simulink model "stm32f0_eep_emulation_demo"  (Simulink 7.3)
settings: Solver=FixedStepDiscrete  SolverMode=SingleTasking  StartTime=0.0  StopTime=10  RelTol=1e-3
PreLoadFcn:
  | waijung.modelPreload; % Required for working with Waijung Blockset. Do not remove.
undefined symbols (not defined in the file): LQFP48, STM32F072CB
libraries: simulink x1, stm32f0_device_config_lib x1
CloseFcn:
  | waijung.modelClose; % Required for working with Waijung Blockset. Do not remove.
settings Model: Creator=Krisada  LastModifiedBy=Krisada
settings OptimizationCC: OptimizeModelRefInitCode=on  LifeSpan=1
settings HardwareCC: ProdEndianess=LittleEndian  ProdHWDeviceType=ARM Compatible->Cortex - M0  TargetEndianess=LittleEndian  TargetHWDeviceType=ARM Compatible->Cortex - M0
settings RTWCC: SystemTargetFile=stm32f0.tlc  GenerateMakefile=off  TemplateMakefile=ert_default_tmf  Description=STM32F0 Target  ProcessScript=stm32f0_make_rtw_hook
settings CodeAppCC: IgnoreCustomStorageClasses=off
settings STFCustomTargetCC: ModelReferenceCompliant=off  CombineOutputUpdateFcns=on  ERTCustomFileBanners=on  SupportContinuousTime=off  SupportNonInlinedSFcns=off  SystemTargetFile=stm32f0.tlc
settings ERTTargetCC: MultiwordLength=2048  ModelReferenceCompliant=off  ParMdlRefBuildCompliant=off  CompOptLevelCompliant=off  ERTFirstTimeCompliant=off  ModelStepFunctionPrototypeControlCompliant=off  CPPClassGenCompliant=off  ExtModeMexFile=noextcomm  InlinedParameterPlacement=NonHierarchical  ERTSrcFileBannerTemplate=stm32f0_code_template.cgt  ERTHdrFileBannerTemplate=stm32f0_code_template.cgt  ERTDataSrcFileTemplate=stm32f0_code_template.cgt  ERTDataHdrFileTemplate=stm32f0_code_template.cgt  ERTCustomFileTemplate=stm32f0_file_process.tlc

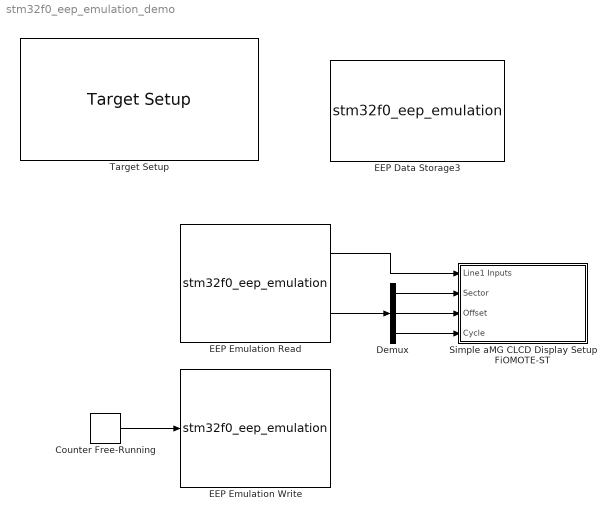
== system stm32f0_eep_emulation_demo ==
  Counter Free-Running : simulink/Sources/Counter Free-Running  SystemSampleTime=-1  NumBits=16  tsamp=-1
  Demux : Demux  Outputs=3
  EEP Data Storage3 : S-Function  FunctionName=stm32f0_eep_emulation  Parameters=conf,inputporttype,inputportwidth,outputporttype,outputportwidth,eepfilename,eepinfo,varname,optionstring,sampletime,blockid  EnableBusSupport=off  mask(stm32f0_eep_emulation){conf=Setup, datatype=uint8, storagedefinename='s', storagename=<empty>, varname='<empty>', initialvalue=8, storageindex=-1, eepfilename='stm32f0_eep_emulation_demo.eeprom', eepinfo='', sampletime=inf, enablecustomportlabel=off, cinputportlabel=0, coutputportlabel=, portpinstr=0, blockid=EEPDataStorage3, inputporttype=[], inputportwidth=[], inputportlabel={}, outputporttype=[], outputportwidth=[], outputportlabel={}, compat=0, optionstring=[]}
      mask prompts: conf "Configuration"; datatype "Storage type"; storagedefinename "Storage name"; storagename "Storage name"; varname "Var name (hidden)"; initialvalue "Initial value"; storageindex "Storage name index (hidden)"; eepfilename "EEP file name (hidden)"; eepinfo "EEP Information (hidden), [name, initialvalue, datatype]"; sampletime "Sample time (sec)"; enablecustomportlabel "Enable custom port labels (Ex. In1, In2, In3)"; cinputportlabel "Custom input port labels (Ex. In1, In2, In3)"; coutputportlabel "Custom output port labels (Ex. Out1, Out2, Out3)"; portpinstr "Port Pin String"; blockid "Block ID"; inputporttype "Input Port Type"; inputportwidth "Input Port Width"; inputportlabel "Input Port Label"; outputporttype "Output Port Type"; outputportwidth "Output Port Width"; outputportlabel "Output port label"; compat "Compatibility (Reserved for future use)"; optionstring "String(s) to be passed to TLC"
      mask init:
      | stm32f0_eep_emulation_callback('init');
      mask Help: web(fullfile(waijungdocroot,'stm32f0_eep_emulation.htm'), '-browser')
      mask StyleString: popup(Setup|Read|Write),popup(double|single|int8|uint8|int16|uint16|int32|uint32),edit,popup(<empty>),edit,edit,edit,edit,edit,edit,checkbox,edit,edit,edit,edit,edit,edit,edit,edit,edit,edit,edit,edit
      mask CallbackString: stm32f0_eep_emulation_callback('conf');||stm32f0_eep_emulation_callback('storagedefinename');||stm32f0_eep_emulation_callback('varname');|||stm32f0_eep_emulation_callback('eepfilename');||stm32f0_eep_emulation_callback('sampletime');|stm32f0_eep_emulation_callback('enablecustomportlabel');|stm32f0_eep_emulation_callback('conf');|stm32f0_eep_emulation_callback('conf');||stm32f0_eep_emulation_callback('blockid');||||||||
      mask Display: text(0.5, 0.5, '[EEP Setup]\nName: s\nType: uint8','ver','middle','hor','center');
  EEP Emulation Read : S-Function  FunctionName=stm32f0_eep_emulation  Parameters=conf,inputporttype,inputportwidth,outputporttype,outputportwidth,eepfilename,eepinfo,varname,optionstring,sampletime,blockid  EnableBusSupport=off  mask(stm32f0_eep_emulation){conf=Read, datatype=single, storagedefinename='Data1,Data2', storagename=s, varname='s', initialvalue=[1.0 2.0], storageindex=0, eepfilename='stm32f0_eep_emulation_demo.eeprom', eepinfo='s,3,8,-', debuginfo=on, sampletime=inf, enablecustomportlabel=off, cinputportlabel=0, coutputportlabel=, portpinstr=0, blockid=EEPEmulationRead, inputporttype=[], inputportwidth=[], inputportlabel={}, outputporttype=[3 6], outputportwidth=[1 3], outputportlabel={'s','Debug'}, compat=0, optionstring=["s","0","3","on","","","","","","","2","s","3","8","dummy","0","0"]}
      mask prompts: conf "Configuration"; datatype "Storage type"; storagedefinename "Storage name"; storagename "Storage name"; varname "Var name (hidden)"; initialvalue "Initial value"; storageindex "Storage name index (hidden)"; eepfilename "EEP file name (hidden)"; eepinfo "EEP Information (hidden), [name, initialvalue, datatype]"; debuginfo "Debug information"; sampletime "Sample time (sec)"; enablecustomportlabel "Enable custom port labels (Ex. In1, In2, In3)"; cinputportlabel "Custom input port labels (Ex. In1, In2, In3)"; coutputportlabel "Custom output port labels (Ex. Out1, Out2, Out3)"; portpinstr "Port Pin String"; blockid "Block ID"; inputporttype "Input Port Type"; inputportwidth "Input Port Width"; inputportlabel "Input Port Label"; outputporttype "Output Port Type"; outputportwidth "Output Port Width"; outputportlabel "Output port label"; compat "Compatibility (Reserved for future use)"; optionstring "String(s) to be passed to TLC"
      mask help: Read a value from EEProm Emulation of the specified variable anme.
      mask init:
      | stm32f0_eep_emulation_callback('init');
      mask Help: web(fullfile(waijungdocroot,'stm32f0_eep_emulation.htm'), '-browser')
      mask StyleString: popup(Setup|Read|Write),popup(double|single|int8|uint8|int16|uint16|int32|uint32),edit,popup(s),edit,edit,edit,edit,edit,checkbox,edit,checkbox,edit,edit,edit,edit,edit,edit,edit,edit,edit,edit,edit,edit
      mask CallbackString: stm32f0_eep_emulation_callback('conf');||stm32f0_eep_emulation_callback('storagedefinename');||stm32f0_eep_emulation_callback('varname');|||stm32f0_eep_emulation_callback('eepfilename');||stm32f0_eep_emulation_callback('debuginfo');|stm32f0_eep_emulation_callback('sampletime');|stm32f0_eep_emulation_callback('enablecustomportlabel');|stm32f0_eep_emulation_callback('conf');|stm32f0_eep_emulation_callback('conf');||stm32f0_eep_emulation_callback('blockid');||||||||
      mask Display: text(0.5, 0.5, '[EEP Read]\nName: s\nTs (sec): 0.01','ver','middle','hor','center'); port_label('output', 1,'s'); port_label('output', 2,'Debug');
  EEP Emulation Write : S-Function  FunctionName=stm32f0_eep_emulation  Parameters=conf,inputporttype,inputportwidth,outputporttype,outputportwidth,eepfilename,eepinfo,varname,optionstring,sampletime,blockid  EnableBusSupport=off  mask(stm32f0_eep_emulation){conf=Write, datatype=single, storagedefinename='Data1,Data2', storagename=s, varname='s', initialvalue=[1.0 2.0], storageindex=0, eepfilename='stm32f0_eep_emulation_demo.eeprom', eepinfo='s,3,8,-', debuginfo=off, sampletime=inf, enablecustomportlabel=off, cinputportlabel=0, coutputportlabel=, portpinstr=0, blockid=EEPEmulationWrite, inputporttype=[-1], inputportwidth=[], inputportlabel={'s'}, outputporttype=[], outputportwidth=[], outputportlabel={}, compat=0, optionstring=["s","0","3","off","","","","","","","2","s","3","8","dummy","0","0"]}
      mask prompts: conf "Configuration"; datatype "Storage type"; storagedefinename "Storage name"; storagename "Storage name"; varname "Var name (hidden)"; initialvalue "Initial value"; storageindex "Storage name index (hidden)"; eepfilename "EEP file name (hidden)"; eepinfo "EEP Information (hidden), [name, initialvalue, datatype]"; debuginfo "Debug information"; sampletime "Sample time (sec)"; enablecustomportlabel "Enable custom port labels (Ex. In1, In2, In3)"; cinputportlabel "Custom input port labels (Ex. In1, In2, In3)"; coutputportlabel "Custom output port labels (Ex. Out1, Out2, Out3)"; portpinstr "Port Pin String"; blockid "Block ID"; inputporttype "Input Port Type"; inputportwidth "Input Port Width"; inputportlabel "Input Port Label"; outputporttype "Output Port Type"; outputportwidth "Output Port Width"; outputportlabel "Output port label"; compat "Compatibility (Reserved for future use)"; optionstring "String(s) to be passed to TLC"
      mask help: Write data value to the specified variable name, to store in EEProm Emulation.
      mask init:
      | stm32f0_eep_emulation_callback('init');
      mask Help: web(fullfile(waijungdocroot,'stm32f0_eep_emulation.htm'), '-browser')
      mask StyleString: popup(Setup|Read|Write),popup(double|single|int8|uint8|int16|uint16|int32|uint32),edit,popup(s),edit,edit,edit,edit,edit,checkbox,edit,checkbox,edit,edit,edit,edit,edit,edit,edit,edit,edit,edit,edit,edit
      mask CallbackString: stm32f0_eep_emulation_callback('conf');||stm32f0_eep_emulation_callback('storagedefinename');||stm32f0_eep_emulation_callback('varname');|||stm32f0_eep_emulation_callback('eepfilename');||stm32f0_eep_emulation_callback('debuginfo');|stm32f0_eep_emulation_callback('sampletime');|stm32f0_eep_emulation_callback('enablecustomportlabel');|stm32f0_eep_emulation_callback('conf');|stm32f0_eep_emulation_callback('conf');||stm32f0_eep_emulation_callback('blockid');||||||||
      mask Display: text(0.5, 0.5, '[EEP Write]\nName: s\nTs (sec): 0.01','ver','middle','hor','center'); port_label('input', 1,'s');
  Simple aMG CLCD Display Setup FiOMOTE-ST : Subsystem
      settings: CopyFcn=set_param(gcbh, 'LinkStatus', 'none')
  Target Setup : stm32f0_device_config_lib/Target Setup  Priority=100  compiler=GNU ARM  previous_compiler=GNU ARM  mcu=STM32F072CB (LQFP48)  mcustr=STM32F072CB  stdlib=STM32F072  clockconfig=FiO MOTE-ST Default (HSEOSC-8MHz/HCLK-48MHz)  system_stm32f0xx_c_path=F:\trunk\targets\stm32f0_target\stm32f0\utils\STM32F0xx_AN4055\stm32f0_default\hse8mhz_pll_hclk48mhz  showmemoryconfiguration=on  stacksize=0x400  heapsize=0  enableautocompiledownload=on  fullchiperase=off  programmerinterface=aMG USB Connect  editctrlstr=on  compilercontrolstr=$(patsubst %, -I%, .) -mcpu=cortex-m0 -mthumb -mabi=aapcs -Wall -O3 -mfloat-abi=soft -ffunction-sections -fdata-sections -fno-strict-aliasing -fno-builtin --short-enums  assemblercontrolstr=$(patsubst %, -I%, .) -mcpu=cortex-m0 -mtune=cortex-m0 -mthumb -Wall -O3 -Wa,-amhls=$(<:.s=.lst) -D__STACK_SIZE=$(STACK_SIZE) -D__HEAP_SIZE=$(HEAP_SIZE)  linkercontrolstr="-T$(LD_SCRIPT) -Wl,-Map=$(MAP),--cref,--no-warn-mismatch -mcpu=cortex-m0 -mthumb  -Wall -O3 -mabi=aapcs -lc -specs=nosys.specs"  runafterdownload=on  execprofile=None  profileruart=3  profilerbaud=500000  profilertxpin=Not used  profilerinitstr=0.01,48000000,480000,500000,0  manualsetsampletime=off  sampletime=0.01  blockid=TargetSetup  systickreloadvalue=480000  hseval=8000000  lastprofileruart=3  hclk=48000000  flashorigin=0x8000000  flashlength=128k  ramorigin=0x20000000  ramlength=16k  useextram=off
  wires:
  Demux/1 -> Simple aMG CLCD Display Setup FiOMOTE-ST/2(Sector)
  Demux/2 -> Simple aMG CLCD Display Setup FiOMOTE-ST/3(Offset)
  Demux/3 -> Simple aMG CLCD Display Setup FiOMOTE-ST/4(Cycle)
  EEP Emulation Read/2 -> Demux/1
  EEP Emulation Read/1 -> Simple aMG CLCD Display Setup FiOMOTE-ST/1(Line1 Inputs)
  Counter Free-Running/1 -> EEP Emulation Write/1

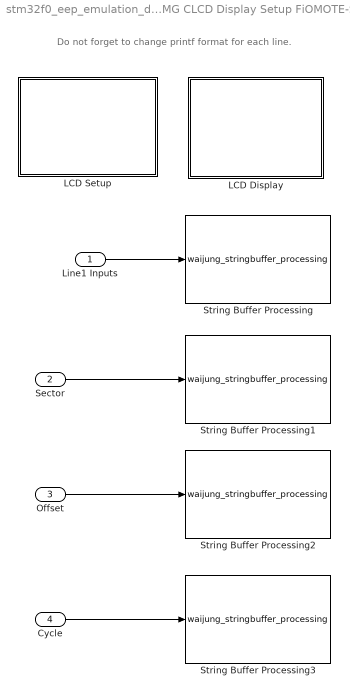
== system stm32f0_eep_emulation_demo/Simple aMG CLCD Display Setup FiOMOTE-ST ==
  note: Do not forget to change printf format for each line.
  Line1 Inputs : Inport  OutDataType=fixdt(1, 16)  OutScaling=2^0
  Sector : Inport  Port=2  OutDataType=fixdt(1, 16)  OutScaling=2^0
  Offset : Inport  Port=3  OutDataType=fixdt(1, 16)  OutScaling=2^0
  Cycle : Inport  Port=4  OutDataType=fixdt(1, 16)  OutScaling=2^0
  LCD Display : Subsystem
  LCD Setup : Subsystem
  String Buffer Processing : S-Function  FunctionName=waijung_stringbuffer_processing  Parameters=configuration,varname,sformat,porttypes,portcount,inputtypearray,outputtypearray,sampletime,sampletimestr,blockid  EnableBusSupport=off  mask(waijung_stringbuffer_processing){configuration=sprintf, storagename=Line1, sformat='%u', enableoutput=off, varname=SimpleaMGCLCDDisplaySetupFiOMOTESTLCDSetupVolatileDataStorage_Line1, inputtypearray=[1 -1], outputtypearray=[0], porttypes=["uint32_t"], portcount=1, sampletime=-1, sampletimestr=0.01, blockid=SimpleaMGCLCDDisplaySetupFiOMOTESTStringBufferProcessing}
      mask prompts: configuration "Function"; storagename "String buffer"; sformat "Printf format"; enableoutput "Enable output status"; varname "Variable name"; inputtypearray "Input type array"; outputtypearray "Output type array"; porttypes "Port type list"; portcount "Port type count"; sampletime "Sample time (sec)"; sampletimestr "Compiled sample time (sec) in string"
      mask help:
      | This block implements string processing, sprintf/ sscanf command.
      | Supported format:
      | %u, %i, %o, %x: uint32
      | %d: int32
      | %e, %g, %f: single
      | %c: int8
      |
      | Status:
      |  0: Failed.
      |  Non-zero: Success.
      mask init:
      | waijung_stringbuffer_processing_callback('init');
      mask Help: web(fullfile(waijungdocroot,'String_Buffer_Processing.htm'))
      mask StyleString: popup(sprintf|sscanf),popup(Line1|Line2|Line3|Line4|<output>),edit,checkbox,edit,edit,edit,edit,edit,edit,edit,edit
      mask CallbackString: waijung_stringbuffer_processing_callback('configuration');||waijung_stringbuffer_processing_callback('sformat');|waijung_stringbuffer_processing_callback('enableoutput');||||||waijung_stringbuffer_processing_callback('sampletime');|waijung_stringbuffer_processing_callback('sampletimestr');|waijung_stringbuffer_processing_callback('blockid');
      mask Display: text(0.5, 0.5, '[ sprintf ]\nBuffer: Line1\nTs (sec): 0.01','ver','middle','hor','center');port_label('input', 1,'%u');
  String Buffer Processing1 : S-Function  FunctionName=waijung_stringbuffer_processing  Parameters=configuration,varname,sformat,porttypes,portcount,inputtypearray,outputtypearray,sampletime,sampletimestr,blockid  EnableBusSupport=off  mask(waijung_stringbuffer_processing){configuration=sprintf, storagename=Line2, sformat='Sector:%d', enableoutput=off, varname=SimpleaMGCLCDDisplaySetupFiOMOTESTLCDSetupVolatileDataStorage1_Line2, inputtypearray=[1 -1], outputtypearray=[0], porttypes=["int32_t"], portcount=1, sampletime=-1, sampletimestr=0.01, blockid=SimpleaMGCLCDDisplaySetupFiOMOTESTStringBufferProcessing1}
      mask prompts: configuration "Function"; storagename "String buffer"; sformat "Printf format"; enableoutput "Enable output status"; varname "Variable name"; inputtypearray "Input type array"; outputtypearray "Output type array"; porttypes "Port type list"; portcount "Port type count"; sampletime "Sample time (sec)"; sampletimestr "Compiled sample time (sec) in string"
      mask help:
      | This block implements string processing, sprintf/ sscanf command.
      | Supported format:
      | %u, %i, %o, %x: uint32
      | %d: int32
      | %e, %g, %f: single
      | %c: int8
      |
      | Status:
      |  0: Failed.
      |  Non-zero: Success.
      mask init:
      | waijung_stringbuffer_processing_callback('init');
      mask Help: web(fullfile(waijungdocroot,'String_Buffer_Processing.htm'))
      mask StyleString: popup(sprintf|sscanf),popup(Line1|Line2|Line3|Line4|<output>),edit,checkbox,edit,edit,edit,edit,edit,edit,edit,edit
      mask CallbackString: waijung_stringbuffer_processing_callback('configuration');||waijung_stringbuffer_processing_callback('sformat');|waijung_stringbuffer_processing_callback('enableoutput');||||||waijung_stringbuffer_processing_callback('sampletime');|waijung_stringbuffer_processing_callback('sampletimestr');|waijung_stringbuffer_processing_callback('blockid');
      mask Display: text(0.5, 0.5, '[ sprintf ]\nBuffer: Line2\nTs (sec): 0.01','ver','middle','hor','center');port_label('input', 1,'%d');
  String Buffer Processing2 : S-Function  FunctionName=waijung_stringbuffer_processing  Parameters=configuration,varname,sformat,porttypes,portcount,inputtypearray,outputtypearray,sampletime,sampletimestr,blockid  EnableBusSupport=off  mask(waijung_stringbuffer_processing){configuration=sprintf, storagename=Line3, sformat='Offset:%d', enableoutput=off, varname=SimpleaMGCLCDDisplaySetupFiOMOTESTLCDSetupVolatileDataStorage2_Line3, inputtypearray=[1 -1], outputtypearray=[0], porttypes=["int32_t"], portcount=1, sampletime=-1, sampletimestr=0.01, blockid=SimpleaMGCLCDDisplaySetupFiOMOTESTStringBufferProcessing2}
      mask prompts: configuration "Function"; storagename "String buffer"; sformat "Printf format"; enableoutput "Enable output status"; varname "Variable name"; inputtypearray "Input type array"; outputtypearray "Output type array"; porttypes "Port type list"; portcount "Port type count"; sampletime "Sample time (sec)"; sampletimestr "Compiled sample time (sec) in string"
      mask help:
      | This block implements string processing, sprintf/ sscanf command.
      | Supported format:
      | %u, %i, %o, %x: uint32
      | %d: int32
      | %e, %g, %f: single
      | %c: int8
      |
      | Status:
      |  0: Failed.
      |  Non-zero: Success.
      mask init:
      | waijung_stringbuffer_processing_callback('init');
      mask Help: web(fullfile(waijungdocroot,'String_Buffer_Processing.htm'))
      mask StyleString: popup(sprintf|sscanf),popup(Line1|Line2|Line3|Line4|<output>),edit,checkbox,edit,edit,edit,edit,edit,edit,edit,edit
      mask CallbackString: waijung_stringbuffer_processing_callback('configuration');||waijung_stringbuffer_processing_callback('sformat');|waijung_stringbuffer_processing_callback('enableoutput');||||||waijung_stringbuffer_processing_callback('sampletime');|waijung_stringbuffer_processing_callback('sampletimestr');|waijung_stringbuffer_processing_callback('blockid');
      mask Display: text(0.5, 0.5, '[ sprintf ]\nBuffer: Line3\nTs (sec): 0.01','ver','middle','hor','center');port_label('input', 1,'%d');
  String Buffer Processing3 : S-Function  FunctionName=waijung_stringbuffer_processing  Parameters=configuration,varname,sformat,porttypes,portcount,inputtypearray,outputtypearray,sampletime,sampletimestr,blockid  EnableBusSupport=off  mask(waijung_stringbuffer_processing){configuration=sprintf, storagename=Line4, sformat='Cycle:%d', enableoutput=off, varname=SimpleaMGCLCDDisplaySetupFiOMOTESTLCDSetupVolatileDataStorage3_Line4, inputtypearray=[1 -1], outputtypearray=[0], porttypes=["int32_t"], portcount=1, sampletime=-1, sampletimestr=0.01, blockid=SimpleaMGCLCDDisplaySetupFiOMOTESTStringBufferProcessing3}
      mask prompts: configuration "Function"; storagename "String buffer"; sformat "Printf format"; enableoutput "Enable output status"; varname "Variable name"; inputtypearray "Input type array"; outputtypearray "Output type array"; porttypes "Port type list"; portcount "Port type count"; sampletime "Sample time (sec)"; sampletimestr "Compiled sample time (sec) in string"
      mask help:
      | This block implements string processing, sprintf/ sscanf command.
      | Supported format:
      | %u, %i, %o, %x: uint32
      | %d: int32
      | %e, %g, %f: single
      | %c: int8
      |
      | Status:
      |  0: Failed.
      |  Non-zero: Success.
      mask init:
      | waijung_stringbuffer_processing_callback('init');
      mask Help: web(fullfile(waijungdocroot,'String_Buffer_Processing.htm'))
      mask StyleString: popup(sprintf|sscanf),popup(Line1|Line2|Line3|Line4|<output>),edit,checkbox,edit,edit,edit,edit,edit,edit,edit,edit
      mask CallbackString: waijung_stringbuffer_processing_callback('configuration');||waijung_stringbuffer_processing_callback('sformat');|waijung_stringbuffer_processing_callback('enableoutput');||||||waijung_stringbuffer_processing_callback('sampletime');|waijung_stringbuffer_processing_callback('sampletimestr');|waijung_stringbuffer_processing_callback('blockid');
      mask Display: text(0.5, 0.5, '[ sprintf ]\nBuffer: Line4\nTs (sec): 0.01','ver','middle','hor','center');port_label('input', 1,'%d');
  wires:
  Line1 Inputs/1 -> String Buffer Processing/1
  Sector/1 -> String Buffer Processing1/1
  Offset/1 -> String Buffer Processing2/1
  Cycle/1 -> String Buffer Processing3/1

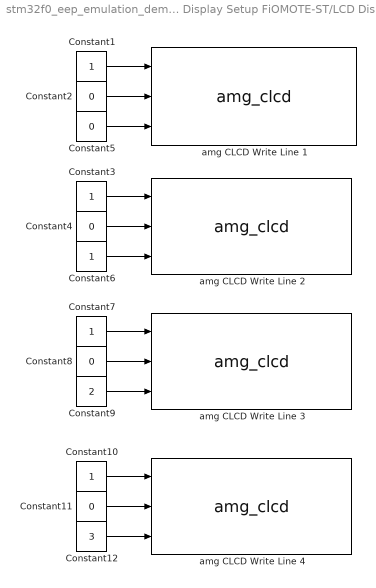
== system stm32f0_eep_emulation_demo/Simple aMG CLCD Display Setup FiOMOTE-ST/LCD Display ==
  Constant{1,3,6..7,10} (5 alike) : Constant  OutDataTypeMode=uint8  OutDataType=fixdt(1, 16)  OutScaling=2^0  OutDataTypeStr=uint8
  Constant{2,4..5,8,11} (5 alike) : Constant  Value=0  OutDataTypeMode=uint8  OutDataType=fixdt(1, 16)  OutScaling=2^0  OutDataTypeStr=uint8
  Constant12 : Constant  Value=3  OutDataTypeMode=uint8  OutDataType=fixdt(1, 16)  OutScaling=2^0  OutDataTypeStr=uint8
  Constant9 : Constant  Value=2  OutDataTypeMode=uint8  OutDataType=fixdt(1, 16)  OutScaling=2^0  OutDataTypeStr=uint8
  amg CLCD Write Line 1 : S-Function  FunctionName=amg_clcd  Parameters=module,configuration,inputtypearray,outputtypearray,confstr,sampletime,sampletimestr,blockid  EnableBusSupport=off  mask(amg_clcd){configuration=Transaction, module=1, model=amg CLCD Std, interface=4-bits, linecount=4, columncount=20, gpiotype=Push-pull, controlport=E, control_rs=15, control_en=11, control_rw=13, dataport=A, data0=7, data1=5, data2=3, data3=1, usestringbuffer=on, stringbuffer=Line1, varname=SimpleaMGCLCDDisplaySetupFiOMOTESTLCDSetupVolatileDataStorage_Line1, inputtypearray=[3 -1 -1 -1], outputtypearray=[0], confstr=["4","4","20","PP","E","15","11","13","","A","","","","","7","5","3","1","1","SimpleaMGCLCDDisplaySetupFiOMOTESTLCDSetupVolatileDataStorage_Line1","1","0","0","0","1","0","0","0","0","stm32f0"], sampletime=0.05, sampletimestr=0.05, blockid=SimpleaMGCLCDDisplaySetupFiOMOTESTLCDDisplayamgCLCDWriteLine1}
      mask prompts: model "LCD model:"; linecount "Number of lines:"; columncount "Number of columns:"; gpiotype "GPIO Pull-Up/Down:"; controlport "GPIO control port:"; control_rs "GPIO control pin, RS:"; control_en "GPIO control pin, EN:"; control_rw "GPIO control pin, RW:"; dataport "GPIO data D[7:4] port"; data0 "GPIO data pin, D4:"; data1 "GPIO data pin, D5:"; data2 "GPIO data pin, D6:"; data3 "GPIO data pin, D7:"; usestringbuffer "Use string buffer"; stringbuffer "String buffer"; varname "Variable name"; inputtypearray "Input type array"; outputtypearray "Output type array"; confstr "Configuration string"; sampletime "Sample time (sec)"; sampletimestr "Compiled sample time (sec) in string"
      mask help:
      | Note for cmd:
      | 1 - Clear LCD Line before write.
      | 0 or otherwise - Write into LCD Line with existing data.
      mask init:
      | amg_clcd_callback('init');
      mask Help: web(fullfile(waijungdocroot,'amg_clcd_write.htm'), '-browser')
      mask StyleString: popup(Setup|Transaction),popup(1|2|3|4),popup(amg CLCD Std),popup(4-bits),edit,edit,popup(Push-pull|Open-drain),popup(A|B|C|D|E|F|G|H|I),popup(0|1|2|3|4|5|6|7|8|9|10|11|12|13|14|15),popup(0|1|2|3|4|5|6|7|8|9|10|11|12|13|14|15),popup(0|1|2|3|4|5|6|7|8|9|10|11|12|13|14|15),popup(A|B|C|D|E|F|G|H|I),popup(0|1|2|3|4|5|6|7|8|9|10|11|12|13|14|15),popup(0|1|2|3|4|5|6|7|8|9|10|11|12|13|14|15),popup(0|1|2|3|4|5|6|7|8|9|10|11|12|13|14|15),popup(0|1|2|3|4|5|6|7|8|9|10|11|12|13|14|15),checkbox,popup(Line1|Line2|Line3|Line4),edit,edit,edit,edit,edit,edit,edit
      mask CallbackString: amg_clcd_callback('configuration');||||||||||||||||amg_clcd_callback('usestringbuffer');||amg_clcd_callback('varname');|||amg_clcd_callback('confstr');|amg_clcd_callback('sampletime');|amg_clcd_callback('sampletimestr');|amg_clcd_callback('blockid');
      mask Display: text(0.5, 0.5, 'Module: CLCD1 (Write)\nBuffer: Line1\nTs (sec): 0.05','ver','middle','hor','center');port_label('input', 1,'cmd');port_label('input', 2,'xpos');port_label('input', 3,'ypos');
  amg CLCD Write Line 2 : S-Function  FunctionName=amg_clcd  Parameters=module,configuration,inputtypearray,outputtypearray,confstr,sampletime,sampletimestr,blockid  EnableBusSupport=off  mask(amg_clcd){configuration=Transaction, module=1, model=amg CLCD Std, interface=4-bits, linecount=4, columncount=20, gpiotype=Push-pull, controlport=E, control_rs=15, control_en=11, control_rw=13, dataport=A, data0=7, data1=5, data2=3, data3=1, usestringbuffer=on, stringbuffer=Line2, varname=SimpleaMGCLCDDisplaySetupFiOMOTESTLCDSetupVolatileDataStorage1_Line2, inputtypearray=[3 -1 -1 -1], outputtypearray=[0], confstr=["4","4","20","PP","E","15","11","13","","A","","","","","7","5","3","1","1","SimpleaMGCLCDDisplaySetupFiOMOTESTLCDSetupVolatileDataStorage1_Line2","1","0","0","0","1","0","0","0","0","stm32f0"], sampletime=0.05, sampletimestr=0.05, blockid=SimpleaMGCLCDDisplaySetupFiOMOTESTLCDDisplayamgCLCDWriteLine2}
      mask prompts: model "LCD model:"; linecount "Number of lines:"; columncount "Number of columns:"; gpiotype "GPIO Pull-Up/Down:"; controlport "GPIO control port:"; control_rs "GPIO control pin, RS:"; control_en "GPIO control pin, EN:"; control_rw "GPIO control pin, RW:"; dataport "GPIO data D[7:4] port"; data0 "GPIO data pin, D4:"; data1 "GPIO data pin, D5:"; data2 "GPIO data pin, D6:"; data3 "GPIO data pin, D7:"; usestringbuffer "Use string buffer"; stringbuffer "String buffer"; varname "Variable name"; inputtypearray "Input type array"; outputtypearray "Output type array"; confstr "Configuration string"; sampletime "Sample time (sec)"; sampletimestr "Compiled sample time (sec) in string"
      mask help:
      | Note for cmd:
      | 1 - Clear LCD Line before write.
      | 0 or otherwise - Write into LCD Line with existing data.
      mask init:
      | amg_clcd_callback('init');
      mask Help: web(fullfile(waijungdocroot,'amg_clcd_write.htm'), '-browser')
      mask StyleString: popup(Setup|Transaction),popup(1|2|3|4),popup(amg CLCD Std),popup(4-bits),edit,edit,popup(Push-pull|Open-drain),popup(A|B|C|D|E|F|G|H|I),popup(0|1|2|3|4|5|6|7|8|9|10|11|12|13|14|15),popup(0|1|2|3|4|5|6|7|8|9|10|11|12|13|14|15),popup(0|1|2|3|4|5|6|7|8|9|10|11|12|13|14|15),popup(A|B|C|D|E|F|G|H|I),popup(0|1|2|3|4|5|6|7|8|9|10|11|12|13|14|15),popup(0|1|2|3|4|5|6|7|8|9|10|11|12|13|14|15),popup(0|1|2|3|4|5|6|7|8|9|10|11|12|13|14|15),popup(0|1|2|3|4|5|6|7|8|9|10|11|12|13|14|15),checkbox,popup(Line1|Line2|Line3|Line4),edit,edit,edit,edit,edit,edit,edit
      mask CallbackString: amg_clcd_callback('configuration');||||||||||||||||amg_clcd_callback('usestringbuffer');||amg_clcd_callback('varname');|||amg_clcd_callback('confstr');|amg_clcd_callback('sampletime');|amg_clcd_callback('sampletimestr');|amg_clcd_callback('blockid');
      mask Display: text(0.5, 0.5, 'Module: CLCD1 (Write)\nBuffer: Line2\nTs (sec): 0.05','ver','middle','hor','center');port_label('input', 1,'cmd');port_label('input', 2,'xpos');port_label('input', 3,'ypos');
  amg CLCD Write Line 3 : S-Function  FunctionName=amg_clcd  Parameters=module,configuration,inputtypearray,outputtypearray,confstr,sampletime,sampletimestr,blockid  EnableBusSupport=off  mask(amg_clcd){configuration=Transaction, module=1, model=amg CLCD Std, interface=4-bits, linecount=4, columncount=20, gpiotype=Push-pull, controlport=E, control_rs=15, control_en=11, control_rw=13, dataport=A, data0=7, data1=5, data2=3, data3=1, usestringbuffer=on, stringbuffer=Line3, varname=SimpleaMGCLCDDisplaySetupFiOMOTESTLCDSetupVolatileDataStorage2_Line3, inputtypearray=[3 -1 -1 -1], outputtypearray=[0], confstr=["4","4","20","PP","E","15","11","13","","A","","","","","7","5","3","1","1","SimpleaMGCLCDDisplaySetupFiOMOTESTLCDSetupVolatileDataStorage2_Line3","1","0","0","0","1","0","0","0","0","stm32f0"], sampletime=0.05, sampletimestr=0.05, blockid=SimpleaMGCLCDDisplaySetupFiOMOTESTLCDDisplayamgCLCDWriteLine3}
      mask prompts: model "LCD model:"; linecount "Number of lines:"; columncount "Number of columns:"; gpiotype "GPIO Pull-Up/Down:"; controlport "GPIO control port:"; control_rs "GPIO control pin, RS:"; control_en "GPIO control pin, EN:"; control_rw "GPIO control pin, RW:"; dataport "GPIO data D[7:4] port"; data0 "GPIO data pin, D4:"; data1 "GPIO data pin, D5:"; data2 "GPIO data pin, D6:"; data3 "GPIO data pin, D7:"; usestringbuffer "Use string buffer"; stringbuffer "String buffer"; varname "Variable name"; inputtypearray "Input type array"; outputtypearray "Output type array"; confstr "Configuration string"; sampletime "Sample time (sec)"; sampletimestr "Compiled sample time (sec) in string"
      mask help:
      | Note for cmd:
      | 1 - Clear LCD Line before write.
      | 0 or otherwise - Write into LCD Line with existing data.
      mask init:
      | amg_clcd_callback('init');
      mask Help: web(fullfile(waijungdocroot,'amg_clcd_write.htm'), '-browser')
      mask StyleString: popup(Setup|Transaction),popup(1|2|3|4),popup(amg CLCD Std),popup(4-bits),edit,edit,popup(Push-pull|Open-drain),popup(A|B|C|D|E|F|G|H|I),popup(0|1|2|3|4|5|6|7|8|9|10|11|12|13|14|15),popup(0|1|2|3|4|5|6|7|8|9|10|11|12|13|14|15),popup(0|1|2|3|4|5|6|7|8|9|10|11|12|13|14|15),popup(A|B|C|D|E|F|G|H|I),popup(0|1|2|3|4|5|6|7|8|9|10|11|12|13|14|15),popup(0|1|2|3|4|5|6|7|8|9|10|11|12|13|14|15),popup(0|1|2|3|4|5|6|7|8|9|10|11|12|13|14|15),popup(0|1|2|3|4|5|6|7|8|9|10|11|12|13|14|15),checkbox,popup(Line1|Line2|Line3|Line4),edit,edit,edit,edit,edit,edit,edit
      mask CallbackString: amg_clcd_callback('configuration');||||||||||||||||amg_clcd_callback('usestringbuffer');||amg_clcd_callback('varname');|||amg_clcd_callback('confstr');|amg_clcd_callback('sampletime');|amg_clcd_callback('sampletimestr');|amg_clcd_callback('blockid');
      mask Display: text(0.5, 0.5, 'Module: CLCD1 (Write)\nBuffer: Line3\nTs (sec): 0.05','ver','middle','hor','center');port_label('input', 1,'cmd');port_label('input', 2,'xpos');port_label('input', 3,'ypos');
  amg CLCD Write Line 4 : S-Function  FunctionName=amg_clcd  Parameters=module,configuration,inputtypearray,outputtypearray,confstr,sampletime,sampletimestr,blockid  EnableBusSupport=off  mask(amg_clcd){configuration=Transaction, module=1, model=amg CLCD Std, interface=4-bits, linecount=4, columncount=20, gpiotype=Push-pull, controlport=E, control_rs=15, control_en=11, control_rw=13, dataport=A, data0=7, data1=5, data2=3, data3=1, usestringbuffer=on, stringbuffer=Line4, varname=SimpleaMGCLCDDisplaySetupFiOMOTESTLCDSetupVolatileDataStorage3_Line4, inputtypearray=[3 -1 -1 -1], outputtypearray=[0], confstr=["4","4","20","PP","E","15","11","13","","A","","","","","7","5","3","1","1","SimpleaMGCLCDDisplaySetupFiOMOTESTLCDSetupVolatileDataStorage3_Line4","1","0","0","0","1","0","0","0","0","stm32f0"], sampletime=0.05, sampletimestr=0.05, blockid=SimpleaMGCLCDDisplaySetupFiOMOTESTLCDDisplayamgCLCDWriteLine4}
      mask prompts: model "LCD model:"; linecount "Number of lines:"; columncount "Number of columns:"; gpiotype "GPIO Pull-Up/Down:"; controlport "GPIO control port:"; control_rs "GPIO control pin, RS:"; control_en "GPIO control pin, EN:"; control_rw "GPIO control pin, RW:"; dataport "GPIO data D[7:4] port"; data0 "GPIO data pin, D4:"; data1 "GPIO data pin, D5:"; data2 "GPIO data pin, D6:"; data3 "GPIO data pin, D7:"; usestringbuffer "Use string buffer"; stringbuffer "String buffer"; varname "Variable name"; inputtypearray "Input type array"; outputtypearray "Output type array"; confstr "Configuration string"; sampletime "Sample time (sec)"; sampletimestr "Compiled sample time (sec) in string"
      mask help:
      | Note for cmd:
      | 1 - Clear LCD Line before write.
      | 0 or otherwise - Write into LCD Line with existing data.
      mask init:
      | amg_clcd_callback('init');
      mask Help: web(fullfile(waijungdocroot,'amg_clcd_write.htm'), '-browser')
      mask StyleString: popup(Setup|Transaction),popup(1|2|3|4),popup(amg CLCD Std),popup(4-bits),edit,edit,popup(Push-pull|Open-drain),popup(A|B|C|D|E|F|G|H|I),popup(0|1|2|3|4|5|6|7|8|9|10|11|12|13|14|15),popup(0|1|2|3|4|5|6|7|8|9|10|11|12|13|14|15),popup(0|1|2|3|4|5|6|7|8|9|10|11|12|13|14|15),popup(A|B|C|D|E|F|G|H|I),popup(0|1|2|3|4|5|6|7|8|9|10|11|12|13|14|15),popup(0|1|2|3|4|5|6|7|8|9|10|11|12|13|14|15),popup(0|1|2|3|4|5|6|7|8|9|10|11|12|13|14|15),popup(0|1|2|3|4|5|6|7|8|9|10|11|12|13|14|15),checkbox,popup(Line1|Line2|Line3|Line4),edit,edit,edit,edit,edit,edit,edit
      mask CallbackString: amg_clcd_callback('configuration');||||||||||||||||amg_clcd_callback('usestringbuffer');||amg_clcd_callback('varname');|||amg_clcd_callback('confstr');|amg_clcd_callback('sampletime');|amg_clcd_callback('sampletimestr');|amg_clcd_callback('blockid');
      mask Display: text(0.5, 0.5, 'Module: CLCD1 (Write)\nBuffer: Line4\nTs (sec): 0.05','ver','middle','hor','center');port_label('input', 1,'cmd');port_label('input', 2,'xpos');port_label('input', 3,'ypos');
  wires:
  Constant1/1 -> amg CLCD Write Line 1/1
  Constant3/1 -> amg CLCD Write Line 2/1
  Constant4/1 -> amg CLCD Write Line 2/2
  Constant2/1 -> amg CLCD Write Line 1/2
  Constant5/1 -> amg CLCD Write Line 1/3
  Constant7/1 -> amg CLCD Write Line 3/1
  Constant8/1 -> amg CLCD Write Line 3/2
  Constant9/1 -> amg CLCD Write Line 3/3
  Constant10/1 -> amg CLCD Write Line 4/1
  Constant11/1 -> amg CLCD Write Line 4/2
  Constant12/1 -> amg CLCD Write Line 4/3
  Constant6/1 -> amg CLCD Write Line 2/3

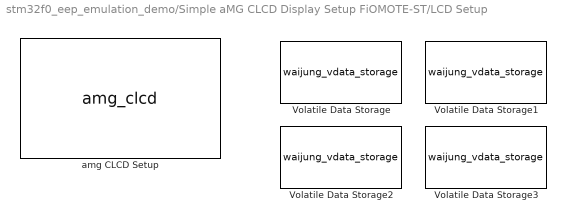
== system stm32f0_eep_emulation_demo/Simple aMG CLCD Display Setup FiOMOTE-ST/LCD Setup ==
  Volatile Data Storage : S-Function  FunctionName=waijung_vdata_storage  Parameters=storagetype,storagename,initval,varname,buffersize,initvalstring,sampletime,sampletimestr,blockid,storagetypestr  EnableBusSupport=off  mask(waijung_vdata_storage){storagetype=string, storagename=Line1, initval=0, varname=SimpleaMGCLCDDisplaySetupFiOMOTESTLCDSetupVolatileDataStorage_Line1, buffersize=64, initvalstring='', webintegration=Disable, weboutputformat='%s', webcgicallback=(void*)0, laststoragetype=string, sampletime=-1, sampletimestr=0.01, blockid=SimpleaMGCLCDDisplaySetupFiOMOTESTLCDSetupVolatileDataStorage, storagetypestr=char}
      mask prompts: storagetype "Storage Type"; storagename "Storage Name (must be a valid variable name)"; initval "Initial value (Apply at Power on Reset only)"; varname "Variable name"; buffersize "Size (bytes)"; initvalstring "Initial value (Apply at Power on Reset only)"; webintegration "Web CGI varget/varset integration"; weboutputformat "Web CGI varget output format"; webcgicallback "Web CGI varset callback"; laststoragetype "Last selected Storage Type"; sampletime "Sample time (sec)"; sampletimestr "Compiled sample time (sec) in string"; storagetypestr "Type string"
      mask help:
      | This block implements a volatile Data Storage.
      |
      | Web CGI varset/varget integratiopn:
      | Enable - In webserver application, allow remote access via http.
      | Disable - Variable is use in local only.
      mask init:
      | waijung_vdata_storage_callback('init');
      mask Help: web(fullfile(waijungdocroot,'Volatile_Data_Storage.htm'))
      mask StyleString: popup(double|single|uint32|int32|uint16|int16|uint8|int8|string),edit,edit,edit,edit,edit,popup(Disable|ReadOnly|Write/ Read|ReadOnly with KeyValuePair|Write/ Read with KeyValuePair),edit,edit,popup(double|single|uint32|int32|uint16|int16|uint8|int8|string),edit,edit,edit,edit
      mask CallbackString: waijung_vdata_storage_callback('storagetype');|waijung_vdata_storage_callback('storagename');|waijung_vdata_storage_callback('initval');|waijung_vdata_storage_callback('varname');||waijung_vdata_storage_callback('initvalstring');|waijung_vdata_storage_callback('webintegration');|waijung_vdata_storage_callback('weboutputformat');|||waijung_vdata_storage_callback('sampletime');|waijung_vdata_storage_callback('sampletimestr');|waijung_vdata_storage_callback('blockid');|
      mask Display: text(0.5, 0.5, 'Name: Line1\nType: string','ver','middle','hor','center')
  Volatile Data Storage1 : S-Function  FunctionName=waijung_vdata_storage  Parameters=storagetype,storagename,initval,varname,buffersize,initvalstring,sampletime,sampletimestr,blockid,storagetypestr  EnableBusSupport=off  mask(waijung_vdata_storage){storagetype=string, storagename=Line2, initval=0, varname=SimpleaMGCLCDDisplaySetupFiOMOTESTLCDSetupVolatileDataStorage1_Line2, buffersize=64, initvalstring='', webintegration=Disable, weboutputformat='%s', webcgicallback=(void*)0, laststoragetype=string, sampletime=-1, sampletimestr=0.01, blockid=SimpleaMGCLCDDisplaySetupFiOMOTESTLCDSetupVolatileDataStorage1, storagetypestr=char}
      mask prompts: storagetype "Storage Type"; storagename "Storage Name (must be a valid variable name)"; initval "Initial value (Apply at Power on Reset only)"; varname "Variable name"; buffersize "Size (bytes)"; initvalstring "Initial value (Apply at Power on Reset only)"; webintegration "Web CGI varget/varset integration"; weboutputformat "Web CGI varget output format"; webcgicallback "Web CGI varset callback"; laststoragetype "Last selected Storage Type"; sampletime "Sample time (sec)"; sampletimestr "Compiled sample time (sec) in string"; storagetypestr "Type string"
      mask help:
      | This block implements a volatile Data Storage.
      |
      | Web CGI varset/varget integratiopn:
      | Enable - In webserver application, allow remote access via http.
      | Disable - Variable is use in local only.
      mask init:
      | waijung_vdata_storage_callback('init');
      mask Help: web(fullfile(waijungdocroot,'Volatile_Data_Storage.htm'))
      mask StyleString: popup(double|single|uint32|int32|uint16|int16|uint8|int8|string),edit,edit,edit,edit,edit,popup(Disable|ReadOnly|Write/ Read|ReadOnly with KeyValuePair|Write/ Read with KeyValuePair),edit,edit,popup(double|single|uint32|int32|uint16|int16|uint8|int8|string),edit,edit,edit,edit
      mask CallbackString: waijung_vdata_storage_callback('storagetype');|waijung_vdata_storage_callback('storagename');|waijung_vdata_storage_callback('initval');|waijung_vdata_storage_callback('varname');||waijung_vdata_storage_callback('initvalstring');|waijung_vdata_storage_callback('webintegration');|waijung_vdata_storage_callback('weboutputformat');|||waijung_vdata_storage_callback('sampletime');|waijung_vdata_storage_callback('sampletimestr');|waijung_vdata_storage_callback('blockid');|
      mask Display: text(0.5, 0.5, 'Name: Line2\nType: string','ver','middle','hor','center')
  Volatile Data Storage2 : S-Function  FunctionName=waijung_vdata_storage  Parameters=storagetype,storagename,initval,varname,buffersize,initvalstring,sampletime,sampletimestr,blockid,storagetypestr  EnableBusSupport=off  mask(waijung_vdata_storage){storagetype=string, storagename=Line3, initval=0, varname=SimpleaMGCLCDDisplaySetupFiOMOTESTLCDSetupVolatileDataStorage2_Line3, buffersize=64, initvalstring='', webintegration=Disable, weboutputformat='%s', webcgicallback=(void*)0, laststoragetype=string, sampletime=-1, sampletimestr=0.01, blockid=SimpleaMGCLCDDisplaySetupFiOMOTESTLCDSetupVolatileDataStorage2, storagetypestr=char}
      mask prompts: storagetype "Storage Type"; storagename "Storage Name (must be a valid variable name)"; initval "Initial value (Apply at Power on Reset only)"; varname "Variable name"; buffersize "Size (bytes)"; initvalstring "Initial value (Apply at Power on Reset only)"; webintegration "Web CGI varget/varset integration"; weboutputformat "Web CGI varget output format"; webcgicallback "Web CGI varset callback"; laststoragetype "Last selected Storage Type"; sampletime "Sample time (sec)"; sampletimestr "Compiled sample time (sec) in string"; storagetypestr "Type string"
      mask help:
      | This block implements a volatile Data Storage.
      |
      | Web CGI varset/varget integratiopn:
      | Enable - In webserver application, allow remote access via http.
      | Disable - Variable is use in local only.
      mask init:
      | waijung_vdata_storage_callback('init');
      mask Help: web(fullfile(waijungdocroot,'Volatile_Data_Storage.htm'))
      mask StyleString: popup(double|single|uint32|int32|uint16|int16|uint8|int8|string),edit,edit,edit,edit,edit,popup(Disable|ReadOnly|Write/ Read|ReadOnly with KeyValuePair|Write/ Read with KeyValuePair),edit,edit,popup(double|single|uint32|int32|uint16|int16|uint8|int8|string),edit,edit,edit,edit
      mask CallbackString: waijung_vdata_storage_callback('storagetype');|waijung_vdata_storage_callback('storagename');|waijung_vdata_storage_callback('initval');|waijung_vdata_storage_callback('varname');||waijung_vdata_storage_callback('initvalstring');|waijung_vdata_storage_callback('webintegration');|waijung_vdata_storage_callback('weboutputformat');|||waijung_vdata_storage_callback('sampletime');|waijung_vdata_storage_callback('sampletimestr');|waijung_vdata_storage_callback('blockid');|
      mask Display: text(0.5, 0.5, 'Name: Line3\nType: string','ver','middle','hor','center')
  Volatile Data Storage3 : S-Function  FunctionName=waijung_vdata_storage  Parameters=storagetype,storagename,initval,varname,buffersize,initvalstring,sampletime,sampletimestr,blockid,storagetypestr  EnableBusSupport=off  mask(waijung_vdata_storage){storagetype=string, storagename=Line4, initval=0, varname=SimpleaMGCLCDDisplaySetupFiOMOTESTLCDSetupVolatileDataStorage3_Line4, buffersize=64, initvalstring='', webintegration=Disable, weboutputformat='%s', webcgicallback=(void*)0, laststoragetype=string, sampletime=-1, sampletimestr=0.01, blockid=SimpleaMGCLCDDisplaySetupFiOMOTESTLCDSetupVolatileDataStorage3, storagetypestr=char}
      mask prompts: storagetype "Storage Type"; storagename "Storage Name (must be a valid variable name)"; initval "Initial value (Apply at Power on Reset only)"; varname "Variable name"; buffersize "Size (bytes)"; initvalstring "Initial value (Apply at Power on Reset only)"; webintegration "Web CGI varget/varset integration"; weboutputformat "Web CGI varget output format"; webcgicallback "Web CGI varset callback"; laststoragetype "Last selected Storage Type"; sampletime "Sample time (sec)"; sampletimestr "Compiled sample time (sec) in string"; storagetypestr "Type string"
      mask help:
      | This block implements a volatile Data Storage.
      |
      | Web CGI varset/varget integratiopn:
      | Enable - In webserver application, allow remote access via http.
      | Disable - Variable is use in local only.
      mask init:
      | waijung_vdata_storage_callback('init');
      mask Help: web(fullfile(waijungdocroot,'Volatile_Data_Storage.htm'))
      mask StyleString: popup(double|single|uint32|int32|uint16|int16|uint8|int8|string),edit,edit,edit,edit,edit,popup(Disable|ReadOnly|Write/ Read|ReadOnly with KeyValuePair|Write/ Read with KeyValuePair),edit,edit,popup(double|single|uint32|int32|uint16|int16|uint8|int8|string),edit,edit,edit,edit
      mask CallbackString: waijung_vdata_storage_callback('storagetype');|waijung_vdata_storage_callback('storagename');|waijung_vdata_storage_callback('initval');|waijung_vdata_storage_callback('varname');||waijung_vdata_storage_callback('initvalstring');|waijung_vdata_storage_callback('webintegration');|waijung_vdata_storage_callback('weboutputformat');|||waijung_vdata_storage_callback('sampletime');|waijung_vdata_storage_callback('sampletimestr');|waijung_vdata_storage_callback('blockid');|
      mask Display: text(0.5, 0.5, 'Name: Line4\nType: string','ver','middle','hor','center')
  amg CLCD Setup : S-Function  FunctionName=amg_clcd  Parameters=module,configuration,inputtypearray,outputtypearray,confstr,sampletime,sampletimestr,blockid  EnableBusSupport=off  mask(amg_clcd){configuration=Setup, module=1, model=amg CLCD Std, interface=4-bits, linecount=4, columncount=16, gpiotype=Push-pull, controlport=B, control_rs=2, control_rw=10, control_en=11, dataport=B, data0=12, data1=13, data2=14, data3=15, usestringbuffer=off, stringbuffer=Line2, varname=clcd_demo_4linesLCDSetupVolatileDataStorage3_Line2, inputtypearray=[0], outputtypearray=[0], confstr=["4","4","16","PP","B","2","11","10","","B","","","","","12","13","14","15","0","","0","1","0","0","0","0","0","0","0","stm32f0"], sampletime=-1, sampletimestr=0.01, blockid=SimpleaMGCLCDDisplaySetupFiOMOTESTLCDSetupamgCLCDSetup}
      mask prompts: model "LCD model:"; linecount "Number of lines:"; columncount "Number of columns:"; gpiotype "GPIO Pull-Up/Down:"; controlport "GPIO control port:"; control_rs "GPIO control pin, RS:"; control_rw "GPIO control pin, RW:"; control_en "GPIO control pin, EN:"; dataport "GPIO data D[7:4] port"; data0 "GPIO data pin, D4:"; data1 "GPIO data pin, D5:"; data2 "GPIO data pin, D6:"; data3 "GPIO data pin, D7:"; usestringbuffer "Use string buffer"; stringbuffer "String buffer"; varname "Variable name"; inputtypearray "Input type array"; outputtypearray "Output type array"; confstr "Configuration string"; sampletime "Sample time (sec)"; sampletimestr "Compiled sample time (sec) in string"
      mask init:
      | amg_clcd_callback('init');
      mask Help: web(fullfile(waijungdocroot,'amg_clcd_setup.htm'), '-browser')
      mask StyleString: popup(Setup|Transaction),popup(1|2|3|4),popup(amg CLCD Std),popup(4-bits),edit,edit,popup(Push-pull|Open-drain),popup(A|B|C|D|E|F|G|H|I),popup(0|1|2|3|4|5|6|7|8|9|10|11|12|13|14|15),popup(0|1|2|3|4|5|6|7|8|9|10|11|12|13|14|15),popup(0|1|2|3|4|5|6|7|8|9|10|11|12|13|14|15),popup(A|B|C|D|E|F|G|H|I),popup(0|1|2|3|4|5|6|7|8|9|10|11|12|13|14|15),popup(0|1|2|3|4|5|6|7|8|9|10|11|12|13|14|15),popup(0|1|2|3|4|5|6|7|8|9|10|11|12|13|14|15),popup(0|1|2|3|4|5|6|7|8|9|10|11|12|13|14|15),checkbox,popup(Line3|Line1|Line2|Line4),edit,edit,edit,edit,edit,edit,edit
      mask CallbackString: amg_clcd_callback('configuration');||||||||||||||||amg_clcd_callback('usestringbuffer');||amg_clcd_callback('varname');|||amg_clcd_callback('confstr');|amg_clcd_callback('sampletime');|amg_clcd_callback('sampletimestr');|amg_clcd_callback('blockid');
      mask Display: text(0.5, 0.5, 'Module: CLCD1 (Setup)\nInterface: 4-bits\nCntrl: B2/B10/B11\nD[7:4]: B12/B13/B14/B15\nTs (sec): 0.01','ver','middle','hor','center');
